simulink model "float_mch_TemplateMatchingContinuous"  (R2020a)
settings: Solver=VariableStepAuto  StartTime=0  StopTime=5  RelTol=1e-3
values from neighbouring files (symbols this model uses):
  score = [3000]    [float_mch_run_TemplateMatchingContinuous.m]
libraries: dspfdesign x2, simulink x2, dspswit3 x1
settings Model: Creator=sbuccelli  LastModifiedBy=diflo

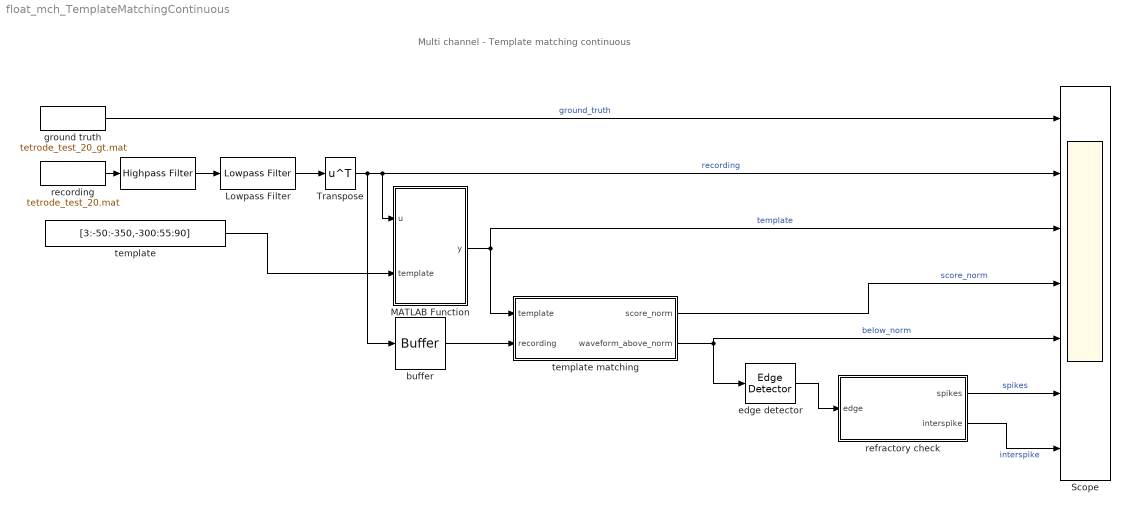
== system float_mch_TemplateMatchingContinuous ==
  note: Multi channel - Template matching continuous
  " " : dspfdesign/Highpass Filter  FilterType=IIR  DesignForMinimumOrder=on  FilterOrder=50  StopbandFrequency=1  PassbandFrequency=300  StopbandAttenuation=80  PassbandRipple=0.1  InheritSampleRate=off  SampleRate=30000  SimulateUsing=Interpreted execution  roundingMode=Floor  coeffsDataTypeStr=fixdt(1,16)
  Lowpass Filter : dspfdesign/Lowpass Filter  FilterType=IIR  DesignForMinimumOrder=on  FilterOrder=3  PassbandFrequency=3500  StopbandFrequency=8500  PassbandRipple=0.1  StopbandAttenuation=80  InheritSampleRate=off  SampleRate=30000  SimulateUsing=Interpreted execution  roundingMode=Floor  coeffsDataTypeStr=fixdt(1,16)
  MATLAB Function : MATLAB Function  TreatAsAtomicUnit=on
  Scope : Scope  NumInputPorts=7
  Transpose : Math  Operator=transpose  SaturateOnIntegerOverflow=on
  buffer : Buffer  N=16  V=15  OutputFrames=off
  edge detector : dspswit3/Edge Detector  InputProcessing=Columns as channels (frame based)
      settings: SourceProductBaseCode=DS
  ground truth : FromFile  FileName=tetrode_test_20_gt.mat  SampleTime=1/30000
  recording : FromFile  FileName=tetrode_test_20.mat  SampleTime=1/30000
  refractory check : Subsystem
  template : Constant  Value=[3:-50:-350,-300:55:90]  SampleTime=1/30000
  template matching : Subsystem
  wires:
  edge detector/1 -> refractory check/1("edge  ")
  refractory check/1(spikes) -> Scope/6  "spikes"
  refractory check/2(interspike) -> Scope/7  "interspike"
  template matching/2(waveform_above_norm) -> Scope/5, edge detector/1  "below_norm"
  buffer/1 -> template matching/2(recording)
  template matching/1(score_norm) -> Scope/4  "score_norm"
  ground truth/1 -> Scope/1  "ground_truth"
  recording/1 -> " "/1
  Transpose/1 -> MATLAB Function/1(u), Scope/2, buffer/1  "recording"
  template/1 -> MATLAB Function/2(template)
  MATLAB Function/1(y) -> Scope/3, template matching/1(template)  "template"
  " "/1 -> Lowpass Filter/1
  Lowpass Filter/1 -> Transpose/1

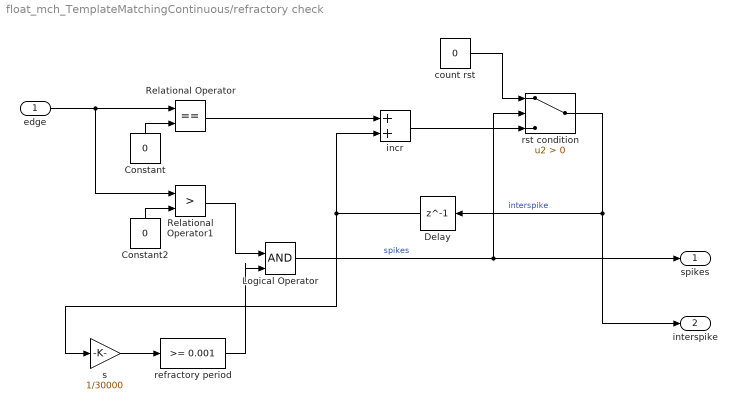
== system float_mch_TemplateMatchingContinuous/refractory check ==
  "edge  " : Inport
  Constant : Constant  Value=0
  Constant2 : Constant  Value=0
  Delay : Delay  DelayLength=1  InitialCondition=1
  Logical Operator : Logic  IconShape=distinctive  AllPortsSameDT=off  OutDataTypeStr=boolean
  Relational Operator : RelationalOperator  Operator===  OutDataTypeStr=boolean  RndMeth=Simplest
  Relational Operator1 : RelationalOperator  Operator=>  OutDataTypeStr=boolean  RndMeth=Simplest
  count rst : Constant  Value=0
  incr : Sum  AccumDataTypeStr=double
  refractory period : simulink/Logic and Bit Operations/Compare To Constant  relop=>=  const=0.001  OutDataTypeStr=boolean
  rst condition : Switch  Criteria=u2 > Threshold  OutDataTypeStr=double
  s : Gain  Gain=1/30000
  spikes : Outport
  interspike : Outport  Port=2
  wires:
  count rst/1 -> rst condition/1
  Constant/1 -> Relational Operator/2
  Constant2/1 -> Relational Operator1/2
  Relational Operator1/1 -> Logical Operator/1
  refractory period/1 -> Logical Operator/2
  Logical Operator/1 -> spikes/1, rst condition/2  "spikes"
  incr/1 -> rst condition/3
  rst condition/1 -> interspike/1, Delay/1  "interspike"
  Delay/1 -> s/1, incr/2
  Relational Operator/1 -> incr/1
  "edge  "/1 -> Relational Operator1/1, Relational Operator/1
  s/1 -> refractory period/1

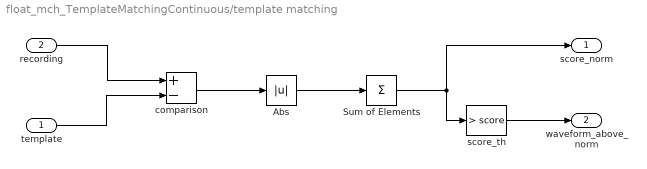
== system float_mch_TemplateMatchingContinuous/template matching ==
  template : Inport
  recording : Inport  Port=2
  Abs : Abs
  Sum of Elements : Sum  Inputs=+  CollapseMode=Specified dimension
  comparison : Sum  Inputs=+-
  score_th : simulink/Logic and Bit Operations/Compare To Constant  relop=>  const=score  OutDataTypeStr=boolean
  score_norm : Outport
  waveform_above_norm : Outport  Port=2
  wires:
  Abs/1 -> Sum of Elements/1
  comparison/1 -> Abs/1
  Sum of Elements/1 -> score_th/1, score_norm/1
  recording/1 -> comparison/1
  score_th/1 -> waveform_above_norm/1
  template/1 -> comparison/2

== matlab function float_mch_TemplateMatchingContinuous/MATLAB Function ==
  data: u input; template input; y output
function y = reptemp(u,template)

y = repmat(template,[1,size(u,2)]);
